simulink model "check_SWC_InpMgmt_AFE"  (R2022b)
settings: configuration reference "DC_DC_Charger_Configuration" (kept outside this file)
values from neighbouring files (symbols this model uses):
  DC_VOLT_ADC_GAIN = 4095/3.3/2    (= 620.454545455)    [ConfigMe_AFE.m]    (also in SWC_InpMgmt_AFE.sldd = 620.454545454545
                
                    
     ; check_SWC_InpMgmt_AFE.sldd = 620.454545454545
                
                    
     )
  DC_VOLT_SNSR_GAIN = 3.3/1000    (= 0.0033)    [ConfigMe_AFE.m]    (also in SWC_InpMgmt_AFE.sldd = 0.0033
                
                    
               ; check_SWC_InpMgmt_AFE.sldd = 0.0033
                
                    
               )
  GRID_CURR_ADC_GAIN = 4096/3.3/2    (= 620.606060606)    [ConfigMe_AFE.m]    (also in SWC_InpMgmt_AFE.sldd = 620.60606060606
                
                    
      ; check_SWC_InpMgmt_AFE.sldd = 620.60606060606
                
                    
      )
  GRID_CURR_SNSR_GAIN = 3.3/50/1.414    (= 0.046676096181)    [ConfigMe_AFE.m]    (also in SWC_InpMgmt_AFE.sldd = 0.0466760961810466
                
                    
   ; check_SWC_InpMgmt_AFE.sldd = 0.0466760961810466
                
                    
   )
  GRID_VOLT_ADC_GAIN = 4095/3.3/2    (= 620.454545455)    [ConfigMe_AFE.m]    (also in SWC_InpMgmt_AFE.sldd = 620.4545455
                
                    
          ; check_SWC_InpMgmt_AFE.sldd = 620.4545455
                
                    
          )
  GRID_VOLT_SNSR_GAIN = 3.3/240/1.414    (= 0.00972418670438)    [ConfigMe_AFE.m]    (also in SWC_InpMgmt_AFE.sldd = 0.009724187
                
                    
          ; check_SWC_InpMgmt_AFE.sldd = 0.009724187
                
                    
          )
libraries: common_lib x20
settings Model: DataDictionary=SWC_InpMgmt_AFE.sldd  SimulationMode=accelerator  ExtModeTrigDuration=8  Creator=E0654638  LastModifiedBy=E0660158
settings ConfigSetRef: SourceName=DC_DC_Charger_Configuration

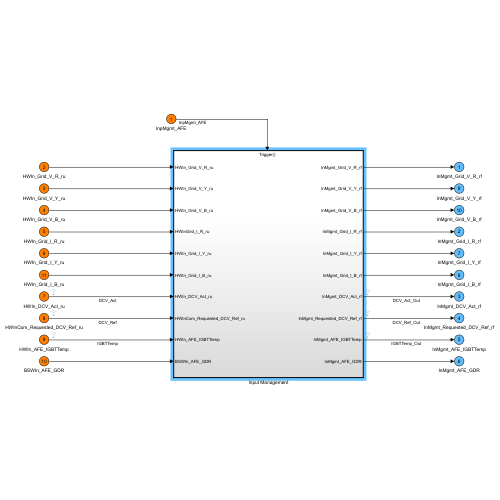
[thumbnail: Simulink's stored preview of the top-level diagram]
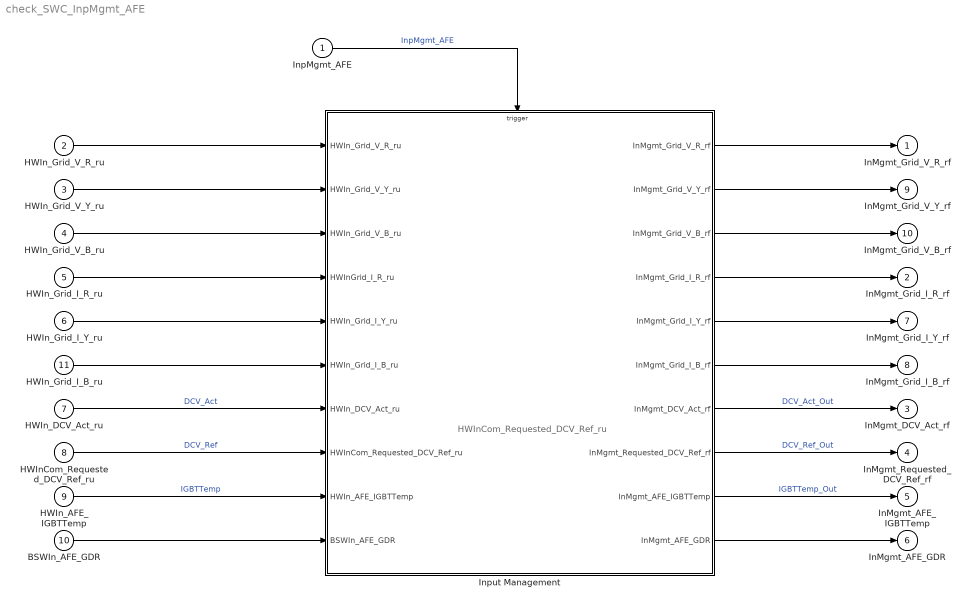
== system check_SWC_InpMgmt_AFE ==
  note: HWInCom_Requested_DCV_Ref_ru
  InpMgmt_AFE : Inport  Description=Inverter HVDC voltage  OutMin=0  OutMax=1000  PortDimensions=1  SampleTime=0.001  OutputFunctionCall=on
  HWIn_Grid_V_R_ru : Inport  Port=2  OutDataTypeStr=uint16
  HWIn_Grid_V_Y_ru : Inport  Port=3  OutDataTypeStr=uint16
  HWIn_Grid_V_B_ru : Inport  Port=4  OutDataTypeStr=uint16
  HWIn_Grid_I_R_ru : Inport  Port=5  OutDataTypeStr=uint16
  HWIn_Grid_I_Y_ru : Inport  Port=6  OutDataTypeStr=uint16
  HWIn_DCV_Act_ru : Inport  Port=7  OutDataTypeStr=uint16
  HWInCom_Requested_DCV_Ref_ru : Inport  Port=8  OutDataTypeStr=uint16
  HWIn_AFE_IGBTTemp : Inport  Port=9  OutDataTypeStr=boolean
  BSWIn_AFE_GDR : Inport  Port=10  OutDataTypeStr=uint16
  HWIn_Grid_I_B_ru : Inport  Port=11  OutDataTypeStr=uint16
  Input Management : Subsystem
  InMgmt_Grid_V_R_rf : Outport  VectorParamsAs1DForOutWhenUnconnected=off
  InMgmt_Grid_I_R_rf : Outport  Port=2  VectorParamsAs1DForOutWhenUnconnected=off
  InMgmt_DCV_Act_rf : Outport  Port=3  OutDataTypeStr=uint16  VectorParamsAs1DForOutWhenUnconnected=off
  InMgmt_Requested_DCV_Ref_rf : Outport  Port=4  OutDataTypeStr=uint16  VectorParamsAs1DForOutWhenUnconnected=off
  InMgmt_AFE_IGBTTemp : Outport  Port=5  OutDataTypeStr=boolean  VectorParamsAs1DForOutWhenUnconnected=off
  InMgmt_AFE_GDR : Outport  Port=6  VectorParamsAs1DForOutWhenUnconnected=off
  InMgmt_Grid_I_Y_rf : Outport  Port=7  VectorParamsAs1DForOutWhenUnconnected=off
  InMgmt_Grid_I_B_rf : Outport  Port=8  VectorParamsAs1DForOutWhenUnconnected=off
  InMgmt_Grid_V_Y_rf : Outport  Port=9  VectorParamsAs1DForOutWhenUnconnected=off
  InMgmt_Grid_V_B_rf : Outport  Port=10  VectorParamsAs1DForOutWhenUnconnected=off
  wires:
  InpMgmt_AFE/1 -> Input Management/Trigger  "InpMgmt_AFE"
  HWIn_DCV_Act_ru/1 -> Input Management/7(HWIn_DCV_Act_ru)  "DCV_Act"
  HWInCom_Requested_DCV_Ref_ru/1 -> Input Management/8(HWInCom_Requested_DCV_Ref_ru)  "DCV_Ref"
  Input Management/8(InMgmt_Requested_DCV_Ref_rf) -> InMgmt_Requested_DCV_Ref_rf/1  "DCV_Ref_Out"
  Input Management/7(InMgmt_DCV_Act_rf) -> InMgmt_DCV_Act_rf/1  "DCV_Act_Out"
  Input Management/1(InMgmt_Grid_V_R_rf) -> InMgmt_Grid_V_R_rf/1
  HWIn_AFE_IGBTTemp/1 -> Input Management/9(HWIn_AFE_IGBTTemp)  "IGBTTemp"
  BSWIn_AFE_GDR/1 -> Input Management/10(BSWIn_AFE_GDR)
  Input Management/10(InMgmt_AFE_GDR) -> InMgmt_AFE_GDR/1
  Input Management/9(InMgmt_AFE_IGBTTemp) -> InMgmt_AFE_IGBTTemp/1  "IGBTTemp_Out"
  HWIn_Grid_I_B_ru/1 -> Input Management/6(HWIn_Grid_I_B_ru)
  HWIn_Grid_I_Y_ru/1 -> Input Management/5(HWIn_Grid_I_Y_ru)
  HWIn_Grid_I_R_ru/1 -> Input Management/4(HWInGrid_I_R_ru)
  HWIn_Grid_V_B_ru/1 -> Input Management/3(HWIn_Grid_V_B_ru)
  HWIn_Grid_V_Y_ru/1 -> Input Management/2(HWIn_Grid_V_Y_ru)
  HWIn_Grid_V_R_ru/1 -> Input Management/1(HWIn_Grid_V_R_ru)
  Input Management/6(InMgmt_Grid_I_B_rf) -> InMgmt_Grid_I_B_rf/1
  Input Management/5(InMgmt_Grid_I_Y_rf) -> InMgmt_Grid_I_Y_rf/1
  Input Management/4(InMgmt_Grid_I_R_rf) -> InMgmt_Grid_I_R_rf/1
  Input Management/2(InMgmt_Grid_V_Y_rf) -> InMgmt_Grid_V_Y_rf/1
  Input Management/3(InMgmt_Grid_V_B_rf) -> InMgmt_Grid_V_B_rf/1

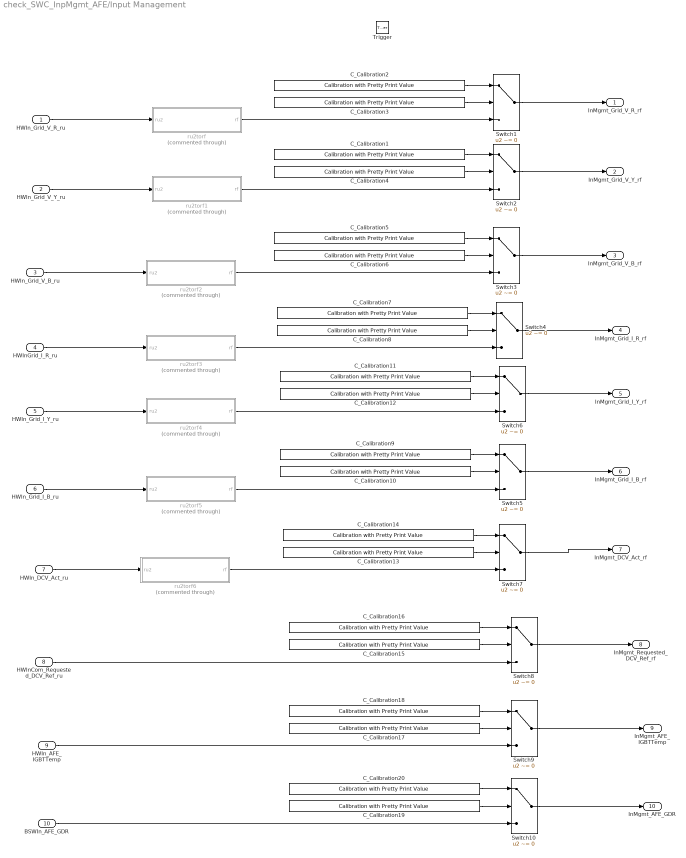
== system check_SWC_InpMgmt_AFE/Input Management ==
  HWIn_Grid_V_R_ru : Inport
  HWIn_Grid_V_Y_ru : Inport  Port=2
  HWIn_Grid_V_B_ru : Inport  Port=3
  HWInGrid_I_R_ru : Inport  Port=4
  HWIn_Grid_I_Y_ru : Inport  Port=5
  HWIn_Grid_I_B_ru : Inport  Port=6
  HWIn_DCV_Act_ru : Inport  Port=7
  HWInCom_Requested_DCV_Ref_ru : Inport  Port=8
  HWIn_AFE_IGBTTemp : Inport  Port=9
  BSWIn_AFE_GDR : Inport  Port=10
  Trigger : TriggerPort  TriggerType=function-call  VariantControl=(inherit)  SampleTimeType=periodic  SampleTime=-1  PortDimensions=1
  C_Calibration1 : common_lib/IO/Calibration with Pretty Print Value  CalValue=InpMgmt_Grid_V_Y_ru2_TC  scaling=None
      settings: SourceProductName=Common Library Blocks
  C_Calibration10 : common_lib/IO/Calibration with Pretty Print Value  CalValue=InpMgmt_Grid_I_B_ru2_TO  scaling=None
      settings: SourceProductName=Common Library Blocks
  C_Calibration11 : common_lib/IO/Calibration with Pretty Print Value  CalValue=InpMgmt_Grid_I_Y_ru2_TC  scaling=None
      settings: SourceProductName=Common Library Blocks
  C_Calibration12 : common_lib/IO/Calibration with Pretty Print Value  CalValue=InpMgmt_Grid_I_Y_ru2_TO  scaling=None
      settings: SourceProductName=Common Library Blocks
  C_Calibration13 : common_lib/IO/Calibration with Pretty Print Value  CalValue=InpMgmt_DCV_Act_ru_TO  scaling=None
      settings: SourceProductName=Common Library Blocks
  C_Calibration14 : common_lib/IO/Calibration with Pretty Print Value  CalValue=InpMgmt_DCV_Act_ru_TC  scaling=None
      settings: SourceProductName=Common Library Blocks
  C_Calibration15 : common_lib/IO/Calibration with Pretty Print Value  CalValue=InpMgmt_Requested_DCV_Ref_ru_TO  scaling=None
      settings: SourceProductName=Common Library Blocks
  C_Calibration16 : common_lib/IO/Calibration with Pretty Print Value  CalValue=InpMgmt_Requested_DCV_Ref_ru_TC  scaling=None
      settings: SourceProductName=Common Library Blocks
  C_Calibration17 : common_lib/IO/Calibration with Pretty Print Value  CalValue=InpMgmt_AFE_IGBTTemp_TO  scaling=None
      settings: SourceProductName=Common Library Blocks
  C_Calibration18 : common_lib/IO/Calibration with Pretty Print Value  CalValue=InpMgmt_AFE_IGBTTemp_TC  scaling=None
      settings: SourceProductName=Common Library Blocks
  C_Calibration19 : common_lib/IO/Calibration with Pretty Print Value  CalValue=InpMgmt_AFE_GDR_TO  scaling=None
      settings: SourceProductName=Common Library Blocks
  C_Calibration2 : common_lib/IO/Calibration with Pretty Print Value  CalValue=InpMgmt_Grid_V_R_ru2_TC  scaling=None
      settings: SourceProductName=Common Library Blocks
  C_Calibration20 : common_lib/IO/Calibration with Pretty Print Value  CalValue=InpMgmt_AFE_GDR_TC  scaling=None
      settings: SourceProductName=Common Library Blocks
  C_Calibration3 : common_lib/IO/Calibration with Pretty Print Value  CalValue=InpMgmt_Grid_V_R_ru2_TO  scaling=None
      settings: SourceProductName=Common Library Blocks
  C_Calibration4 : common_lib/IO/Calibration with Pretty Print Value  CalValue=InpMgmt_Grid_V_Y_ru2_TO  scaling=None
      settings: SourceProductName=Common Library Blocks
  C_Calibration5 : common_lib/IO/Calibration with Pretty Print Value  CalValue=InpMgmt_Grid_V_B_ru2_TC  scaling=None
      settings: SourceProductName=Common Library Blocks
  C_Calibration6 : common_lib/IO/Calibration with Pretty Print Value  CalValue=InpMgmt_Grid_V_B_ru2_TO  scaling=None
      settings: SourceProductName=Common Library Blocks
  C_Calibration7 : common_lib/IO/Calibration with Pretty Print Value  CalValue=InpMgmt_Grid_I_R_ru2_TC  scaling=None
      settings: SourceProductName=Common Library Blocks
  C_Calibration8 : common_lib/IO/Calibration with Pretty Print Value  CalValue=InpMgmt_Grid_I_R_ru2_TO  scaling=None
      settings: SourceProductName=Common Library Blocks
  C_Calibration9 : common_lib/IO/Calibration with Pretty Print Value  CalValue=InpMgmt_Grid_I_B_ru2_TC  scaling=None
      settings: SourceProductName=Common Library Blocks
  Switch{1..10} (10 alike) : Switch  Criteria=u2 ~= 0  SaturateOnIntegerOverflow=off  InputSameDT=off
  ru2torf : Subsystem  Commented=through  mask{Offset_Value=2048, Gain_Value=GRID_VOLT_SNSR_GAIN*GRID_VOLT_ADC_GAIN}
      mask DialogControl ParameterGroupVar Prompt: Offset
      mask DialogControl ParameterGroupVar_copy Prompt: Gain
  ru2torf1 : Subsystem  Commented=through  mask{Offset_Value=2048, Gain_Value=GRID_VOLT_SNSR_GAIN*GRID_VOLT_ADC_GAIN}
      mask DialogControl ParameterGroupVar Prompt: Offset
      mask DialogControl ParameterGroupVar_copy Prompt: Gain
  ru2torf2 : Subsystem  Commented=through  mask{Offset_Value=2048, Gain_Value=GRID_VOLT_SNSR_GAIN*GRID_VOLT_ADC_GAIN}
      mask DialogControl ParameterGroupVar Prompt: Offset
      mask DialogControl ParameterGroupVar_copy Prompt: Gain
  ru2torf3 : Subsystem  Commented=through  mask{Offset_Value=2048, Gain_Value=GRID_CURR_SNSR_GAIN*GRID_CURR_ADC_GAIN}
      mask DialogControl ParameterGroupVar Prompt: Offset
      mask DialogControl ParameterGroupVar_copy Prompt: Gain
  ru2torf4 : Subsystem  Commented=through  mask{Offset_Value=2048, Gain_Value=GRID_CURR_SNSR_GAIN*GRID_CURR_ADC_GAIN}
      mask DialogControl ParameterGroupVar Prompt: Offset
      mask DialogControl ParameterGroupVar_copy Prompt: Gain
  ru2torf5 : Subsystem  Commented=through  mask{Offset_Value=2048, Gain_Value=GRID_CURR_SNSR_GAIN*GRID_CURR_ADC_GAIN}
      mask DialogControl ParameterGroupVar Prompt: Offset
      mask DialogControl ParameterGroupVar_copy Prompt: Gain
  ru2torf6 : Subsystem  Commented=through  mask{Offset_Value=0, Gain_Value=DC_VOLT_ADC_GAIN*DC_VOLT_SNSR_GAIN}
      mask DialogControl ParameterGroupVar Prompt: Offset
      mask DialogControl ParameterGroupVar_copy Prompt: Gain
  InMgmt_Grid_V_R_rf : Outport  OutDataTypeStr=single
  InMgmt_Grid_V_Y_rf : Outport  Port=2  OutDataTypeStr=single
  InMgmt_Grid_V_B_rf : Outport  Port=3  OutDataTypeStr=single
  InMgmt_Grid_I_R_rf : Outport  Port=4  OutDataTypeStr=single
  InMgmt_Grid_I_Y_rf : Outport  Port=5  OutDataTypeStr=single
  InMgmt_Grid_I_B_rf : Outport  Port=6  OutDataTypeStr=single
  InMgmt_DCV_Act_rf : Outport  Port=7
  InMgmt_Requested_DCV_Ref_rf : Outport  Port=8
  InMgmt_AFE_IGBTTemp : Outport  Port=9
  InMgmt_AFE_GDR : Outport  Port=10  OutDataTypeStr=single
  wires:
  HWIn_Grid_I_Y_ru/1 -> ru2torf4/1(ru2)
  HWInGrid_I_R_ru/1 -> ru2torf3/1(ru2)
  HWIn_Grid_I_B_ru/1 -> ru2torf5/1(ru2)
  C_Calibration2/1 -> Switch1/1
  C_Calibration3/1 -> Switch1/2
  ru2torf/1(rf) -> Switch1/3
  Switch2/1 -> InMgmt_Grid_V_Y_rf/1
  ru2torf1/1(rf) -> Switch2/3
  C_Calibration4/1 -> Switch2/2
  C_Calibration1/1 -> Switch2/1
  C_Calibration5/1 -> Switch3/1
  C_Calibration6/1 -> Switch3/2
  ru2torf2/1(rf) -> Switch3/3
  Switch3/1 -> InMgmt_Grid_V_B_rf/1
  Switch4/1 -> InMgmt_Grid_I_R_rf/1
  ru2torf3/1(rf) -> Switch4/3
  C_Calibration8/1 -> Switch4/2
  C_Calibration7/1 -> Switch4/1
  C_Calibration9/1 -> Switch5/1
  C_Calibration10/1 -> Switch5/2
  ru2torf5/1(rf) -> Switch5/3
  Switch5/1 -> InMgmt_Grid_I_B_rf/1
  C_Calibration11/1 -> Switch6/1
  C_Calibration12/1 -> Switch6/2
  ru2torf4/1(rf) -> Switch6/3
  Switch6/1 -> InMgmt_Grid_I_Y_rf/1
  Switch7/1 -> InMgmt_DCV_Act_rf/1
  HWIn_DCV_Act_ru/1 -> ru2torf6/1(ru2)
  C_Calibration13/1 -> Switch7/2
  C_Calibration14/1 -> Switch7/1
  C_Calibration16/1 -> Switch8/1
  C_Calibration15/1 -> Switch8/2
  HWInCom_Requested_DCV_Ref_ru/1 -> Switch8/3
  Switch8/1 -> InMgmt_Requested_DCV_Ref_rf/1
  Switch10/1 -> InMgmt_AFE_GDR/1
  Switch9/1 -> InMgmt_AFE_IGBTTemp/1
  BSWIn_AFE_GDR/1 -> Switch10/3
  HWIn_AFE_IGBTTemp/1 -> Switch9/3
  C_Calibration17/1 -> Switch9/2
  C_Calibration18/1 -> Switch9/1
  C_Calibration19/1 -> Switch10/2
  C_Calibration20/1 -> Switch10/1
  HWIn_Grid_V_R_ru/1 -> ru2torf/1(ru2)
  HWIn_Grid_V_Y_ru/1 -> ru2torf1/1(ru2)
  HWIn_Grid_V_B_ru/1 -> ru2torf2/1(ru2)
  Switch1/1 -> InMgmt_Grid_V_R_rf/1
  ru2torf6/1(rf) -> Switch7/3

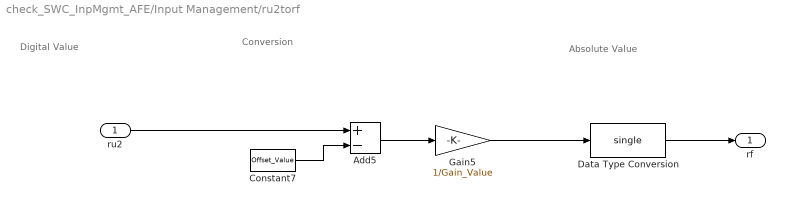
== system check_SWC_InpMgmt_AFE/Input Management/ru2torf ==
  note: Digital Value
  note: Absolute Value
  note: Conversion
  ru2 : Inport
  Add5 : Sum  Inputs=+-
  Constant7 : Constant  Value=Offset_Value
  Data Type Conversion : DataTypeConversion  OutDataTypeStr=single  SaturateOnIntegerOverflow=off  RndMeth=Floor
  Gain5 : Gain  Gain=1/Gain_Value
  rf : Outport  OutDataTypeStr=single
  wires:
  Gain5/1 -> Data Type Conversion/1
  Add5/1 -> Gain5/1
  ru2/1 -> Add5/1
  Constant7/1 -> Add5/2
  Data Type Conversion/1 -> rf/1

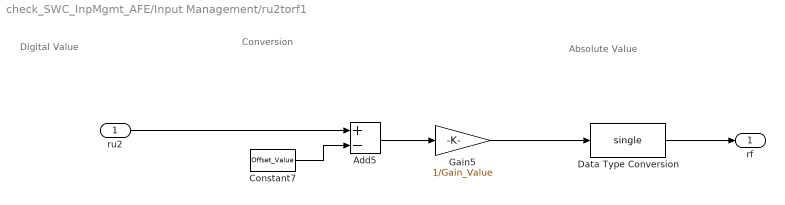
== system check_SWC_InpMgmt_AFE/Input Management/ru2torf1 ==
  note: Digital Value
  note: Absolute Value
  note: Conversion
  ru2 : Inport
  Add5 : Sum  Inputs=+-
  Constant7 : Constant  Value=Offset_Value
  Data Type Conversion : DataTypeConversion  OutDataTypeStr=single  SaturateOnIntegerOverflow=off  RndMeth=Floor
  Gain5 : Gain  Gain=1/Gain_Value
  rf : Outport  OutDataTypeStr=single
  wires:
  Gain5/1 -> Data Type Conversion/1
  Add5/1 -> Gain5/1
  ru2/1 -> Add5/1
  Constant7/1 -> Add5/2
  Data Type Conversion/1 -> rf/1

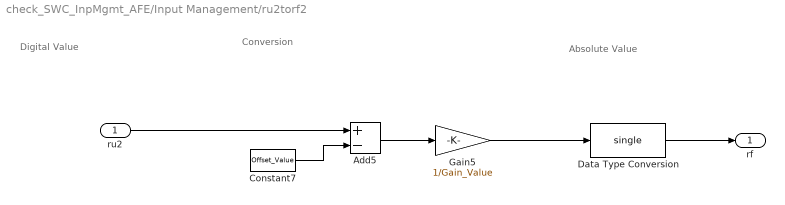
== system check_SWC_InpMgmt_AFE/Input Management/ru2torf2 ==
  note: Digital Value
  note: Absolute Value
  note: Conversion
  ru2 : Inport
  Add5 : Sum  Inputs=+-
  Constant7 : Constant  Value=Offset_Value
  Data Type Conversion : DataTypeConversion  OutDataTypeStr=single  SaturateOnIntegerOverflow=off  RndMeth=Floor
  Gain5 : Gain  Gain=1/Gain_Value
  rf : Outport  OutDataTypeStr=single
  wires:
  Gain5/1 -> Data Type Conversion/1
  Add5/1 -> Gain5/1
  ru2/1 -> Add5/1
  Constant7/1 -> Add5/2
  Data Type Conversion/1 -> rf/1

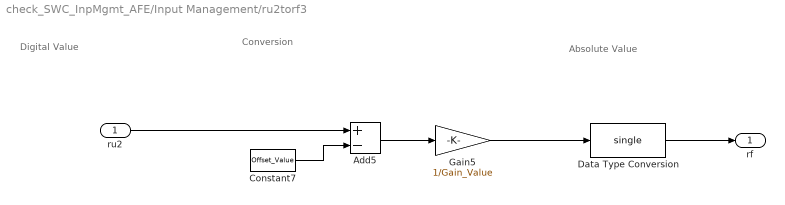
== system check_SWC_InpMgmt_AFE/Input Management/ru2torf3 ==
  note: Digital Value
  note: Absolute Value
  note: Conversion
  ru2 : Inport
  Add5 : Sum  Inputs=+-
  Constant7 : Constant  Value=Offset_Value
  Data Type Conversion : DataTypeConversion  OutDataTypeStr=single  SaturateOnIntegerOverflow=off  RndMeth=Floor
  Gain5 : Gain  Gain=1/Gain_Value
  rf : Outport  OutDataTypeStr=single
  wires:
  Gain5/1 -> Data Type Conversion/1
  Add5/1 -> Gain5/1
  ru2/1 -> Add5/1
  Constant7/1 -> Add5/2
  Data Type Conversion/1 -> rf/1

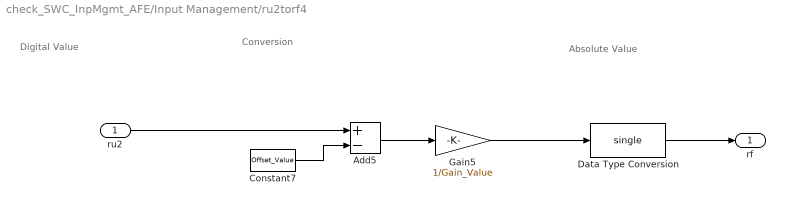
== system check_SWC_InpMgmt_AFE/Input Management/ru2torf4 ==
  note: Digital Value
  note: Absolute Value
  note: Conversion
  ru2 : Inport
  Add5 : Sum  Inputs=+-
  Constant7 : Constant  Value=Offset_Value
  Data Type Conversion : DataTypeConversion  OutDataTypeStr=single  SaturateOnIntegerOverflow=off  RndMeth=Floor
  Gain5 : Gain  Gain=1/Gain_Value
  rf : Outport  OutDataTypeStr=single
  wires:
  Gain5/1 -> Data Type Conversion/1
  Add5/1 -> Gain5/1
  ru2/1 -> Add5/1
  Constant7/1 -> Add5/2
  Data Type Conversion/1 -> rf/1

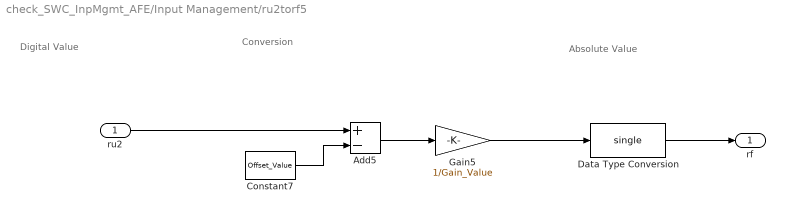
== system check_SWC_InpMgmt_AFE/Input Management/ru2torf5 ==
  note: Digital Value
  note: Absolute Value
  note: Conversion
  ru2 : Inport
  Add5 : Sum  Inputs=+-
  Constant7 : Constant  Value=Offset_Value
  Data Type Conversion : DataTypeConversion  OutDataTypeStr=single  SaturateOnIntegerOverflow=off  RndMeth=Floor
  Gain5 : Gain  Gain=1/Gain_Value
  rf : Outport  OutDataTypeStr=single
  wires:
  Gain5/1 -> Data Type Conversion/1
  Add5/1 -> Gain5/1
  ru2/1 -> Add5/1
  Constant7/1 -> Add5/2
  Data Type Conversion/1 -> rf/1

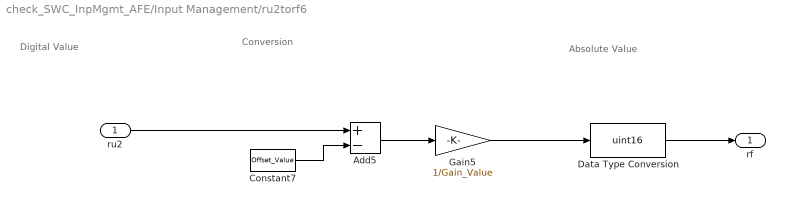
== system check_SWC_InpMgmt_AFE/Input Management/ru2torf6 ==
  note: Digital Value
  note: Absolute Value
  note: Conversion
  ru2 : Inport
  Add5 : Sum  Inputs=+-
  Constant7 : Constant  Value=Offset_Value
  Data Type Conversion : DataTypeConversion  OutDataTypeStr=uint16  SaturateOnIntegerOverflow=off  RndMeth=Floor
  Gain5 : Gain  Gain=1/Gain_Value
  rf : Outport
  wires:
  Gain5/1 -> Data Type Conversion/1
  Add5/1 -> Gain5/1
  ru2/1 -> Add5/1
  Constant7/1 -> Add5/2
  Data Type Conversion/1 -> rf/1
